simulink library "LIB_ORB"  (Simulink 8.8)
settings: Solver=ode45  StartTime=0.0  StopTime=10.0  RelTol=1e-3  EnableMultiTasking=on
undefined symbols (not defined in the file or in its folder): zero_tol
undefined symbols (not defined in the file): CONSTANTS_par
settings Model: Creator=alger  LastModifiedBy=alger

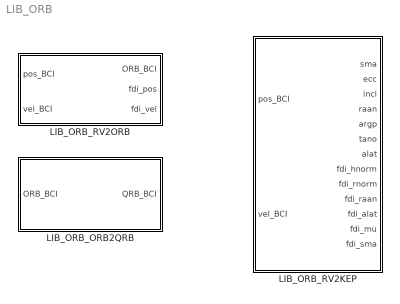
== system LIB_ORB ==
  LIB_ORB_ORB2QRB : Subsystem  TreatAsAtomicUnit=on  mask(Matrix Inverse){}
      mask help:
      | Description:
      |   Performs the conversion of rotation matrix ORB_BCI to rotation matrix
      |   QRB_BCI. the QRB frame when converted to a 3-2-1 rpy sequence is
      |   similar to typical roll pitch and yaw.
      |
      |   The QRB frame is defined as:
      |   QRB frame x-axis is the same as the orbit tangential
      |   QRB frame y-axis is the negative of the orbit normal
      |   QRB frame z-axis is the negative of the orbit radial
      |
      | Inputs:
      |   ORB_BCI  Rotation Matrix ORB_BCI
      |
      | Outputs:
      |   QRB_BCI  Rotation Matrix QRB_BCI
      |
      | uses orb2qrb() function
  LIB_ORB_RV2KEP : Subsystem  TreatAsAtomicUnit=on  mask(Compute Keplarian elements from  postion and velocity){zero_tol=CONSTANTS_par.zero_tol, mu_cst=CONSTANTS_par.mu_earth}
      mask prompts: zero_tol "Near zero tolerence"; mu_cst "Standard gravitational parameter of the primary body (m^3*s-2)"
      mask help:
      | Computes keplarian elements from position and velocity  (intended for plots)
      |
      |
      | Inputs:
      |  pos_BCI: position expressed in a Body Centered Inertial frame  	[m]
      |  vel_BCI: velocity expressed in a Body Centered Inertial frame 	[m/s]
      |
      | Outputs:
      |    sma         Semi-major axis                              		[m]
      |    ecc         eccentricity of orbit        			[-]
      |    incl        Inclination                                  		[rad
      |    raan        Right-ascension of the ascending node        	[rad]
      |    argp        Argument of periapis                     	    	[rad]
      |    tano        true anonmoly                                		[rad]
      |    fdi_hmod_i  Mathematical exception due to hmod = 0        	[1/0]
      |    fdi_rmod_i  Mathematical exception due to rmod = 0        	[1/0]
      |    fdi_raan_i  Mathematical exception in computation of RAAN 	[1/0]
      |    fdi_alat_i  Mathematical exception in computation of alat 	[1/0]
      |    fdi_mu_i    Mathematical exception due to invalid mu_cst  	[1/0]
      |    fdi_sma_i   Mathematical exception in compuattion of sma  	[1/0]
      |
      | uses the rv2kep() function
  LIB_ORB_RV2ORB : Subsystem  TreatAsAtomicUnit=on  mask(Compute Orbital frame){tol=zero_tol}
      mask prompts: tol "Near zero tolerence"
      mask help:
      | Computes Orbitial frame from position and velocity
      |
      | The orbital frame is defined as:
      |   ORB frame x-axis is the orbit radial unit vector)
      |   ORB frame y-axis is the orbit tangential unit vector)
      |   ORB frame z-axis is the orbit normal unit vector)
      |
      | Inputs:
      |  pos_BCI: position expressed in a Body Centered Inertial frame  [m]
      |  vel_BCI: velocity expressed in a Body Centered Inertial frame [m/s]
      |
      | Outputs:
      |  ORB_BCI: rotation matrix relating frame in BCI to ORB
      |  fdi_pos:  fdi indicating norm of pos_BCI is less than zero tolerance
      |  fdi_vel:  fdi indicating norm of pos_BCI is less than zero tolerance
      |
      | uses the rv2orb() function

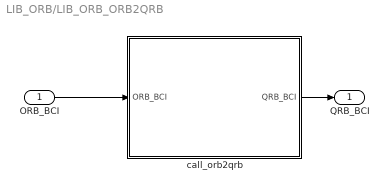
== system LIB_ORB/LIB_ORB_ORB2QRB ==
  ORB_BCI : Inport  PortDimensions=[3,3]
  call_orb2qrb : MATLAB Function  TreatAsAtomicUnit=on
  QRB_BCI : Outport  PortDimensions=[3,3]
  wires:
  ORB_BCI/1 -> call_orb2qrb/1(ORB_BCI)
  call_orb2qrb/1(QRB_BCI) -> QRB_BCI/1

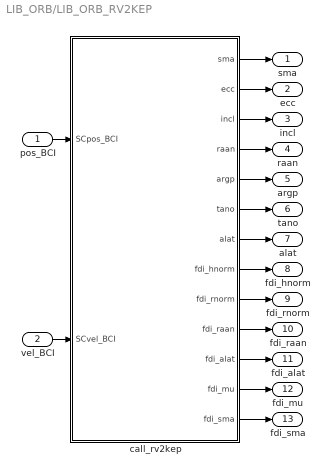
== system LIB_ORB/LIB_ORB_RV2KEP ==
  pos_BCI : Inport  PortDimensions=3
  vel_BCI : Inport  Port=2  PortDimensions=3
  call_rv2kep : MATLAB Function  TreatAsAtomicUnit=on
  sma : Outport  PortDimensions=1
  ecc : Outport  Port=2  PortDimensions=1
  incl : Outport  Port=3  PortDimensions=1
  raan : Outport  Port=4  PortDimensions=1
  argp : Outport  Port=5  PortDimensions=1
  tano : Outport  Port=6  PortDimensions=1
  alat : Outport  Port=7  PortDimensions=1
  fdi_hnorm : Outport  Port=8  PortDimensions=1
  fdi_rnorm : Outport  Port=9  PortDimensions=1
  fdi_raan : Outport  Port=10  PortDimensions=1
  fdi_alat : Outport  Port=11  PortDimensions=1
  fdi_mu : Outport  Port=12  PortDimensions=1
  fdi_sma : Outport  Port=13  PortDimensions=1
  wires:
  call_rv2kep/13(fdi_sma) -> fdi_sma/1
  call_rv2kep/9(fdi_rnorm) -> fdi_rnorm/1
  call_rv2kep/11(fdi_alat) -> fdi_alat/1
  call_rv2kep/10(fdi_raan) -> fdi_raan/1
  call_rv2kep/12(fdi_mu) -> fdi_mu/1
  call_rv2kep/6(tano) -> tano/1
  call_rv2kep/7(alat) -> alat/1
  call_rv2kep/8(fdi_hnorm) -> fdi_hnorm/1
  call_rv2kep/5(argp) -> argp/1
  call_rv2kep/4(raan) -> raan/1
  call_rv2kep/3(incl) -> incl/1
  call_rv2kep/2(ecc) -> ecc/1
  call_rv2kep/1(sma) -> sma/1
  pos_BCI/1 -> call_rv2kep/1(SCpos_BCI)
  vel_BCI/1 -> call_rv2kep/2(SCvel_BCI)

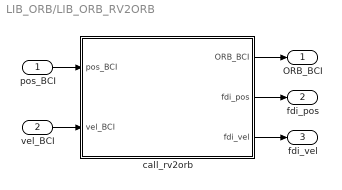
== system LIB_ORB/LIB_ORB_RV2ORB ==
  pos_BCI : Inport  PortDimensions=3
  vel_BCI : Inport  Port=2  PortDimensions=3
  call_rv2orb : MATLAB Function  TreatAsAtomicUnit=on
  ORB_BCI : Outport  PortDimensions=[3,3]
  fdi_pos : Outport  Port=2  PortDimensions=1
  fdi_vel : Outport  Port=3  PortDimensions=1
  wires:
  call_rv2orb/2(fdi_pos) -> fdi_pos/1
  pos_BCI/1 -> call_rv2orb/1(pos_BCI)
  call_rv2orb/1(ORB_BCI) -> ORB_BCI/1
  call_rv2orb/3(fdi_vel) -> fdi_vel/1
  vel_BCI/1 -> call_rv2orb/2(vel_BCI)

== matlab function LIB_ORB_ORB2QRB/call_orb2qrb ==
  data: ORB_BCI input double; QRB_BCI output double
function QRB_BCI  = call_orb2qrb(ORB_BCI)
  %#codegen
  [QRB_BCI] = orb2qrb(ORB_BCI);
end

== matlab function LIB_ORB_RV2ORB/call_rv2orb ==
  data: pos_BCI input double; ORB_BCI output double; vel_BCI input double; fdi_pos output double; tol parameter double; fdi_vel output double
function [ORB_BCI, fdi_pos, fdi_vel] = call_rv2orb(pos_BCI, vel_BCI, tol)
  %#codegen
  [ORB_BCI, fdi_pos, fdi_vel] = rv2orb(pos_BCI, vel_BCI, tol);
end

== matlab function LIB_ORB_RV2KEP/call_rv2kep ==
  data: SCpos_BCI input double size=3; sma output double size=1; SCvel_BCI input double size=3; ecc output double size=1; mu_cst parameter double size=1; incl output double size=1; raan output double size=1; argp output double size=1; tano output double size=1; alat output double size=1; fdi_hnorm output double size=1; fdi_rnorm output double size=1; fdi_raan output double size=1; fdi_alat output double size=1; fdi_mu output double size=1; fdi_sma output double size=1; zero_tol parameter double size=1
function [sma, ecc, incl, raan, argp, tano, alat,    ...
    fdi_hnorm, fdi_rnorm, fdi_raan,   ...
    fdi_alat, fdi_mu,   fdi_sma]   = call_rv2kep(SCpos_BCI, SCvel_BCI, mu_cst, zero_tol)
  %#codegen
  [sma, ecc, incl, raan, argp, tano, alat,    ...
    fdi_hnorm, fdi_rnorm, fdi_raan,   ...
    fdi_alat, fdi_mu,   fdi_sma]        ...
    = rv2kep(SCpos_BCI, SCvel_BCI, mu_cst, zero_tol);
end
